simulink model "openloop_vf_test"  (R2023b)
settings: Solver=FixedStepAuto  StartTime=0.0  StopTime=2  FixedStep=simcfg.Ts_power  RelTol=1e-3
InitFcn:
  | motor_control_params
undefined symbols (not defined in the file or in its folder): inverter, motor, openloop, simcfg
libraries: mcbplantlib x1, autolibpmsmexterior x1, simulink x1
settings Model: Creator=user  LastModifiedBy=user

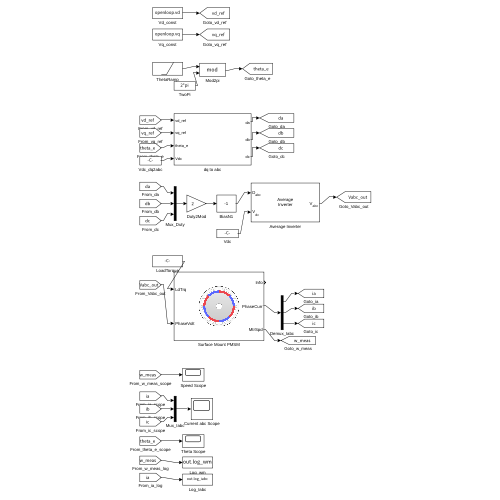
[thumbnail: Simulink's stored preview of the top-level diagram]
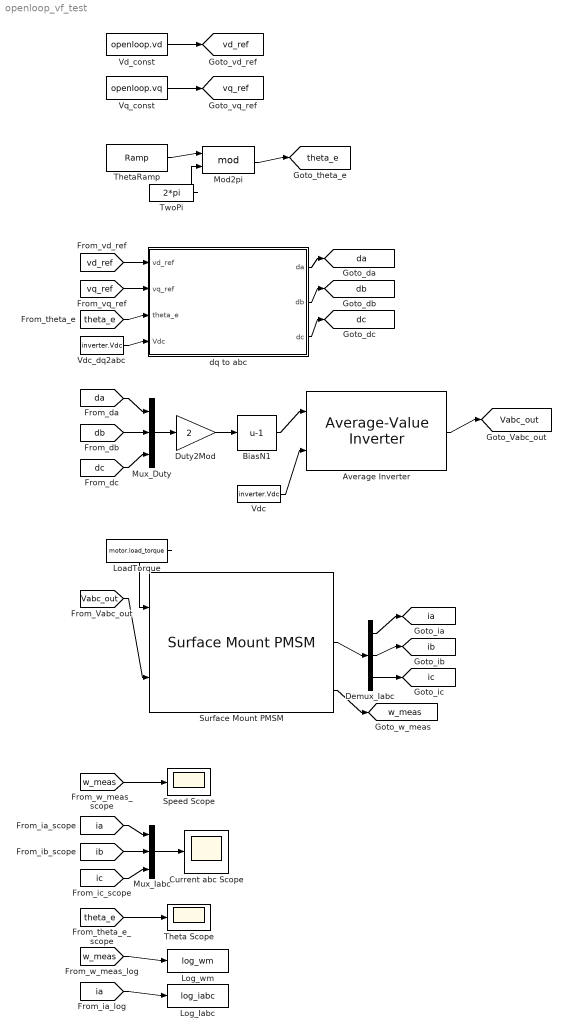
== system openloop_vf_test ==
  Average Inverter : mcbplantlib/Average-Value Inverter
  BiasN1 : Bias  Bias=-1  SaturateOnIntegerOverflow=off
  Current abc Scope : Scope
  Demux_Iabc : Demux  Outputs=3
  Duty2Mod : Gain  Gain=2
  LoadTorque : Constant  Value=motor.load_torque
  Log_Iabc : ToWorkspace  VariableName=log_iabc  SaveFormat=Timeseries  SampleTime=-1
  Log_wm : ToWorkspace  VariableName=log_wm  SaveFormat=Timeseries  SampleTime=-1
  Mod2pi : Math  Operator=mod
  Mux_Duty : Mux  Inputs=3
  Mux_Iabc : Mux  Inputs=3
  Speed Scope : Scope
  Surface Mount PMSM : autolibpmsmexterior/Surface Mount PMSM  port_config=Torque  sim_type=Discrete  Ts=simcfg.Ts_power  P=motor.pole_pairs  Rs=motor.Rs  Ldq_=motor.Ld  KConstText=Permanent flux linkage constant (lambda_pm):  lambda_pm=motor.psi_f  Ke=159.9771  Kt=1.323  mechanical=[motor.J, motor.B, 0]  idq0=[0 0]  theta_init=0  omega_init=0  KConst=motor.psi_f  lambda_pm_calc=motor.psi_f  RefBlkName='autolibpmsmexterior/Surface Mount PMSM'  aMode=5  Ldq="[0.0017      0.0017]"
  Theta Scope : Scope
  ThetaRamp : simulink/Sources/Ramp  slope=2*pi*openloop.freq_hz  start=0  InitialOutput=0
  TwoPi : Constant  Value=2*pi
  Vd_const : Constant  Value=openloop.vd
  Vdc : Constant  Value=inverter.Vdc
  Vdc_dq2abc : Constant  Value=inverter.Vdc
  Vq_const : Constant  Value=openloop.vq
  dq to abc : Subsystem
  tag scope: Vabc_out=global, da=global, db=global, dc=global, ia=global, ib=global, ic=global, theta_e=global, vd_ref=global, vq_ref=global, w_meas=global
  wires:
  Vd_const/1 -> [vd_ref]
  Vq_const/1 -> [vq_ref]
  ThetaRamp/1 -> Mod2pi/1
  TwoPi/1 -> Mod2pi/2
  Mod2pi/1 -> [theta_e]
  [vd_ref] -> dq to abc/1(vd_ref)
  [vq_ref] -> dq to abc/2(vq_ref)
  [theta_e] -> dq to abc/3(theta_e)
  Vdc_dq2abc/1 -> dq to abc/4(Vdc)
  dq to abc/1(da) -> [da]
  dq to abc/2(db) -> [db]
  dq to abc/3(dc) -> [dc]
  [da] -> Mux_Duty/1
  [db] -> Mux_Duty/2
  [dc] -> Mux_Duty/3
  Mux_Duty/1 -> Duty2Mod/1
  Duty2Mod/1 -> BiasN1/1
  BiasN1/1 -> Average Inverter/1
  Vdc/1 -> Average Inverter/2
  Average Inverter/1 -> [Vabc_out]
  LoadTorque/1 -> Surface Mount PMSM/1
  [Vabc_out] -> Surface Mount PMSM/2
  Surface Mount PMSM/2 -> Demux_Iabc/1
  Demux_Iabc/1 -> [ia]
  Demux_Iabc/2 -> [ib]
  Demux_Iabc/3 -> [ic]
  Surface Mount PMSM/3 -> [w_meas]
  [w_meas] -> Speed Scope/1
  [ia] -> Mux_Iabc/1
  [ib] -> Mux_Iabc/2
  [ic] -> Mux_Iabc/3
  Mux_Iabc/1 -> Current abc Scope/1
  [theta_e] -> Theta Scope/1
  [w_meas] -> Log_wm/1
  [ia] -> Log_Iabc/1

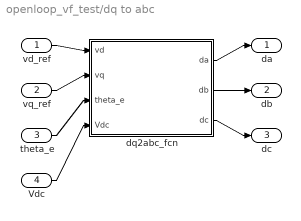
== system openloop_vf_test/dq to abc ==
  vd_ref : Inport
  vq_ref : Inport  Port=2
  theta_e : Inport  Port=3
  Vdc : Inport  Port=4
  dq2abc_fcn : MATLAB Function  TreatAsAtomicUnit=on
  da : Outport
  db : Outport  Port=2
  dc : Outport  Port=3
  wires:
  vd_ref/1 -> dq2abc_fcn/1(vd)
  vq_ref/1 -> dq2abc_fcn/2(vq)
  theta_e/1 -> dq2abc_fcn/3(theta_e)
  Vdc/1 -> dq2abc_fcn/4(Vdc)
  dq2abc_fcn/1(da) -> da/1
  dq2abc_fcn/2(db) -> db/1
  dq2abc_fcn/3(dc) -> dc/1

== matlab function openloop_vf_test/dq to abc/dq2abc_fcn ==
  data: vd input; da output; vq input; theta_e input; Vdc input; db output; dc output
function [da, db, dc] = dq2abc_fcn(vd, vq, theta_e, Vdc)
% dq → 占空比: 逆Park + 逆Clarke + SVPWM + 归一化

% 1. 逆Park: dq → αβ
v_alpha = vd * cos(theta_e) - vq * sin(theta_e);
v_beta  = vd * sin(theta_e) + vq * cos(theta_e);

% 2. 逆Clarke: αβ → abc
va = v_alpha;
vb = -0.5 * v_alpha + sqrt(3)/2 * v_beta;
vc = -0.5 * v_alpha - sqrt(3)/2 * v_beta;

% 3. SVPWM零序注入
v_max = max(max(va, vb), vc);
v_min = min(min(va, vb), vc);
v_n0  = -0.5 * (v_max + v_min);
va = va + v_n0;
vb = vb + v_n0;
vc = vc + v_n0;

% 4. 占空比 [-1,+1] → [0,1]
da = va / Vdc + 0.5;
db = vb / Vdc + 0.5;
dc = vc / Vdc + 0.5;
